simulink model "MMAN3200_2020_PID_PlantPendulum"  (Simulink 8.4)
settings: Solver=ode45  SolverMode=SingleTasking  StartTime=0.0  StopTime=200  RelTol=1e-3
libraries: simulink x2
settings Model: Creator=joseG  LastModifiedBy=joseG
settings OptimizationCC: BlockReduction=off  BooleanDataType=off
settings DebuggingCC: SaveWithParameterizedLinksMsg=none  SignalResolutionControl=TryResolveAllWithWarning  SolverPrmCheckMsg=none  MultiTaskDSMMsg=warning  MultiTaskCondExecSysMsg=none  FcnCallInpInsideContextMsg=EnableAllAsWarning
settings HardwareCC: TargetUnknown=on
settings RTWCC: IncludeERTFirstTime=on
settings GRTTargetCC: CombineOutputUpdateFcns=on  GRTInterface=off

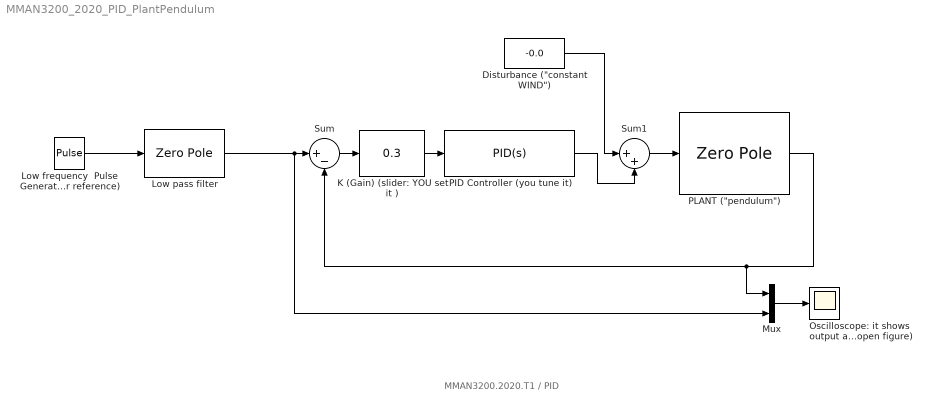
== system MMAN3200_2020_PID_PlantPendulum ==
  note: MMAN3200.2020.T1 / PID
  "Disturbance (\"constant WIND\")" : Constant  Value=-0.0
  K (Gain) (slider: YOU set it ) : simulink/Math Operations/Slider Gain  low=0.3  gain=0.3  high=100
  Low frequency  Pulse Generator (our reference) : DiscretePulseGenerator  PulseType=Time based  Period=80  PulseWidth=50
  Low pass filter : ZeroPole  Tag=PLANT1  Description=PLANT  Zeros=[]  Poles=[-10]  Gain=10
  Mux : Mux  Inputs=2
  "Oscilloscope: it shows output and reference (set-point)  (double-click on icon, once, to open figure)" : Scope
      settings: TimeRange=200  YMin=-0.2  YMax=1.2  MaxDataPoints=500000
  PID Controller (you tune it) : simulink/Continuous/PID Controller  Controller=PID  TimeDomain=Continuous-time  SampleTime=-1  IntegratorMethod=Forward Euler  FilterMethod=Forward Euler  Form=Ideal  P=1  I=0  D=0  N=20  InitialConditionSource=internal  InitialConditionForIntegrator=0  InitialConditionForFilter=0  ExternalReset=none  LimitOutput=on  UpperSaturationLimit=20000  LowerSaturationLimit=-20000  LinearizeAsGain=on  AntiWindupMode=none  Kb=1  TrackingMode=off  Kt=1  PParamMin=[]  PParamMax=[]  IParamMin=[]  IParamMax=[]  DParamMin=[]  DParamMax=[]  NParamMin=[]  NParamMax=[]  KbParamMin=[]  KbParamMax=[]  KtParamMin=[]  KtParamMax=[]  POutMin=[]  POutMax=[]  IOutMin=[]  IOutMax=[]  DOutMin=[]  DOutMax=[]  NOutMin=[]  NOutMax=[]  KbOutMin=[]  KbOutMax=[]  KtOutMin=[]  KtOutMax=[]  IntegratorOutMin=[]  IntegratorOutMax=[]  FilterOutMin=[]  FilterOutMax=[]  SumOutMin=[]  SumOutMax=[]  SumI1OutMin=[]  SumI1OutMax=[]  SumI2OutMin=[]  SumI2OutMax=[]  SumI3OutMin=[]  SumI3OutMax=[]  SumDOutMin=[]  SumDOutMax=[]  SaturationOutMin=[]  SaturationOutMax=[]  IntegratorContinuousStateAttributes=''  IntegratorStateMustResolveToSignalObject=off  IntegratorRTWStateStorageClass=Auto  FilterContinuousStateAttributes=''  FilterStateMustResolveToSignalObject=off  FilterRTWStateStorageClass=Auto  DifferentiatorICPrevScaledInput=0  DifferentiatorOutMin=[]  DifferentiatorOutMax=[]  UseFilter=on
  "PLANT (\"pendulum\")" : ZeroPole  Tag=PLANT1  Description=PLANT  Zeros=[]  Poles="[ -0.5+2i,  -0.5-2i]"  Gain=4.25
  Sum : Sum  Inputs=|+-
  Sum1 : Sum  Inputs=|++
  wires:
  "PLANT (\"pendulum\")"/1 -> Mux/1, Sum/2
  Low pass filter/1 -> Mux/2, Sum/1
  Sum/1 -> K (Gain) (slider: YOU set it )/1
  K (Gain) (slider: YOU set it )/1 -> PID Controller (you tune it)/1
  Mux/1 -> "Oscilloscope: it shows output and reference (set-point)  (double-click on icon, once, to open figure)"/1
  PID Controller (you tune it)/1 -> Sum1/2
  Sum1/1 -> "PLANT (\"pendulum\")"/1
  "Disturbance (\"constant WIND\")"/1 -> Sum1/1
  Low frequency  Pulse Generator (our reference)/1 -> Low pass filter/1
